simulink model "Control_PI_reg_AntiWindup"  (R2020a)
settings: Solver=FixedStepAuto  StartTime=0.0  StopTime=inf  FixedStep=Ts  RelTol=1e-3
undefined symbols (not defined in the file or in its folder): Td, Ti, Zr
libraries: heater_lib x1, simulink x1
settings Model: EnablePacing=on  Creator=MK  LastModifiedBy=olive

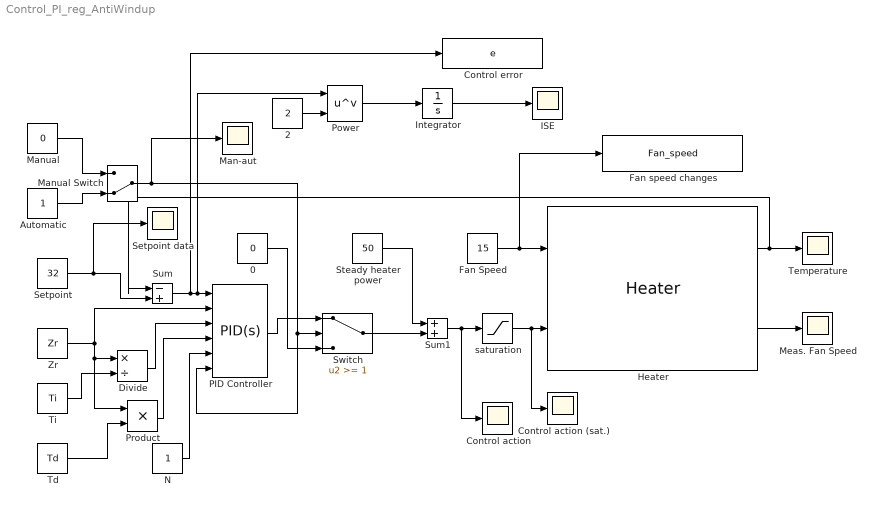
== system Control_PI_reg_AntiWindup ==
  0 : Constant  Value=0
  2 : Constant  Value=2
  Automatic : Constant
  Control action : Scope
  Control action (sat.) : Scope
  Control error : ToWorkspace  VariableName=e  SampleTime=-1
  Divide : Product  Inputs=*/
  Fan Speed : Constant  Value=15
  Fan speed changes : ToWorkspace  VariableName=Fan_speed  SaveFormat=Timeseries  SampleTime=-1
  Heater : heater_lib/Heater  SystemSampleTime=-1  SSRTWFcnClass=[]  Latency=0  AutoFrameSizeCalculation=off
  ISE : Scope
  Integrator : Integrator
  Man-aut : Scope
  Manual : Constant  Value=0
  Manual Switch : ManualSwitch  CurrentSetting=0
  Meas. Fan Speed : Scope
  N : Constant
  PID Controller : simulink/Continuous/PID Controller  Controller=PID  Form=Parallel  TimeDomain=Continuous-time  UseExternalTs=off  SampleTime=-1  IntegratorMethod=Forward Euler  FilterMethod=Forward Euler  ControllerParametersSource=external  P=Zr  I=Zr/Ti  D=Zr*Td  UseFilter=on  N=100  TunerSelectOption=Transfer Function Based (PID Tuner App)  InitialConditionSource=internal  InitialConditionForIntegrator=0  InitialConditionForFilter=0  DifferentiatorICPrevScaledInput=0  ExternalReset=rising  TrackingMode=off  Kt=1  LimitOutput=on  UpperSaturationLimit=50  LowerSaturationLimit=-50  LinearizeAsGain=on  AntiWindupMode=clamping  Kb=0.01  POutMin=[]  POutMax=[]  IOutMin=[]  IOutMax=[]  DOutMin=[]  DOutMax=[]  NOutMin=[]  NOutMax=[]  SumOutMin=[]  SumOutMax=[]  SaturationOutMin=[]  SaturationOutMax=[]  PParamMin=[]  PParamMax=[]  IParamMin=[]  IParamMax=[]  DParamMin=[]  DParamMax=[]  NParamMin=[]  NParamMax=[]  KbParamMin=[]  KbParamMax=[]  KtParamMin=[]  KtParamMax=[]  KbOutMin=[]  KbOutMax=[]  KtOutMin=[]  KtOutMax=[]  IntegratorOutMin=[]  IntegratorOutMax=[]  FilterOutMin=[]  FilterOutMax=[]  SumI1OutMin=[]  SumI1OutMax=[]  SumI2OutMin=[]  SumI2OutMax=[]  SumI3OutMin=[]  SumI3OutMax=[]  SumI4OutMin=[]  SumI4OutMax=[]  SumDOutMin=[]  SumDOutMax=[]  DifferentiatorOutMin=[]  DifferentiatorOutMax=[]  FilterDiffOutCoefMin=[]  FilterDiffOutCoefMax=[]  ReciprocalOutMin=[]  ReciprocalOutMax=[]  SumDenOutMin=[]  SumDenOutMax=[]  SumNumOutMin=[]  SumNumOutMax=[]  DivideOutMin=[]  DivideOutMax=[]  UdiffTsProdOutMin=[]  UdiffTsProdOutMax=[]  NTsProdOutMin=[]  NTsProdOutMax=[]  UintegralTsProdOutMin=[]  UintegralTsProdOutMax=[]  UngainTsProdOutMin=[]  UngainTsProdOutMax=[]  IntegratorContinuousStateAttributes=''  IntegratorStateMustResolveToSignalObject=off  IntegratorRTWStateStorageClass=Auto  FilterContinuousStateAttributes=''  FilterStateMustResolveToSignalObject=off  FilterRTWStateStorageClass=Auto  ParallelPVariant=ExternalParameters  IdealPVariant=Disabled  IVariant=ExternalParameters  DVariant=ExternalParameters  IntegratorVariant=Continuous  SatVariant=Enabled  AWVariant=ContClampingParallel  PCopyVariant=Disabled  TRVariant=Disabled  FdbkBlocksVariant=Forward  IdealPFdbkVariant=Disabled  SatFdbkVariant=Disabled  DerivativeFilterVariant=ContFilter  NVariant=ExternalParameters  NCopyVariant=Disabled  FilterICVariant=InternalICsFilter  IntegratorICVariant=InternalICs  ExternalResetVariant=ExternalReset  TRSumVariant=Passthrough  SumFdbkVariant=Disabled  SumVariant=Sum_PID  TsampFilterVariant=InternalTs  TsampNgainVariant=Passthrough  TsampIntegralVariant=Passthrough
  Power : Math  Operator=pow  SaturateOnIntegerOverflow=on
  Product : Product
  Setpoint : Constant  Value=32
  Setpoint data : Scope
  Steady heater power : Constant  Value=50
  Sum : Sum  Inputs=|-+
  Sum1 : Sum  Inputs=|++
  Switch : Switch  Threshold=1
  Td : Constant  Value=Td
  Temperature : Scope
  Ti : Constant  Value=Ti
  Zr : Constant  Value=Zr
  saturation : Saturate  UpperLimit=100  LowerLimit=0
  wires:
  Heater/1 -> Temperature/1, Sum/1
  Heater/2 -> Meas. Fan Speed/1
  Fan Speed/1 -> Fan speed changes/1, Heater/1
  Zr/1 -> PID Controller/2, Product/1, Divide/1
  Product/1 -> PID Controller/4
  Ti/1 -> Divide/2
  N/1 -> PID Controller/5
  Td/1 -> Product/2
  Divide/1 -> PID Controller/3
  Sum/1 -> Control error/1, Power/1, PID Controller/1
  PID Controller/1 -> Switch/1
  Sum1/1 -> Control action/1, saturation/1
  Steady heater power/1 -> Sum1/1
  saturation/1 -> Control action (sat.)/1, Heater/2
  Setpoint/1 -> Sum/2, Setpoint data/1
  Switch/1 -> Sum1/2
  Manual/1 -> Manual Switch/1
  Manual Switch/1 -> PID Controller/6, Switch/2, Man-aut/1
  Automatic/1 -> Manual Switch/2
  0/1 -> Switch/3
  Integrator/1 -> ISE/1
  Power/1 -> Integrator/1
  2/1 -> Power/2
